simulink model "RequirementsTable"  (R2022b)
settings: Solver=FixedStepAuto  StartTime=0.0  StopTime=10.0  FixedStep=1e-3  RelTol=1e-3  EnableMultiTasking=on
settings Model: DVExtractedSubsystem=Requirements Table  Creator=TheCoaler  LastModifiedBy=TheCoaler
settings SolverCC: AlgebraicLoopSolver=TrustRegion
settings OptimizationCC: EnhancedBackFolding=on  PassReuseOutputArgsAs=Individual arguments  ZeroExternalMemoryAtStartup=off  ZeroInternalMemoryAtStartup=off  MaxStackSize=64  OptimizeBlockOrder=speed  DifferentSizesBufferReuse=on  OptimizationCustomize=off  EfficientTunableParamExpr=on
settings DebuggingCC: ParameterTunabilityLossMsg=error  UnconnectedInputMsg=warning  UnconnectedOutputMsg=warning  UnconnectedLineMsg=warning  FrameProcessingCompatibilityMsg=none  SFMachineParentedDataDiag=warning
settings HardwareCC: ProdBitPerPointer=32  ProdBitPerSizeT=32  ProdBitPerPtrDiffT=32  ProdLargestAtomicInteger=Long  ProdLargestAtomicFloat=Double  ProdWordSize=32  ProdHWDeviceType=ARM Compatible->ARM Cortex
settings ModelReferenceCC: EnableRefExpFcnMdlSchedulingChecks=on
settings SFSimCC: MATLABDynamicMemAlloc=off
settings RTWCC: Description=Embedded Coder  SystemTargetFile=ert.tlc  HardwareBoard=NXP FRDM-K64F  TemplateMakefile=ert_default_tmf  Toolchain=GNU Tools for ARM Embedded Processors
settings CodeAppCC: ForceParamTrailComments=on  IgnoreCustomStorageClasses=off  OperatorAnnotations=on  SimulinkDataObjDesc=on  SFDataObjDesc=on  InsertBlockDesc=on
settings ERTTargetCC: ExtMode=on  ExtModeTransport=4  ExtModeMexFile=sendToCommService  ExtModeMexArgs='RA_Modes' 0

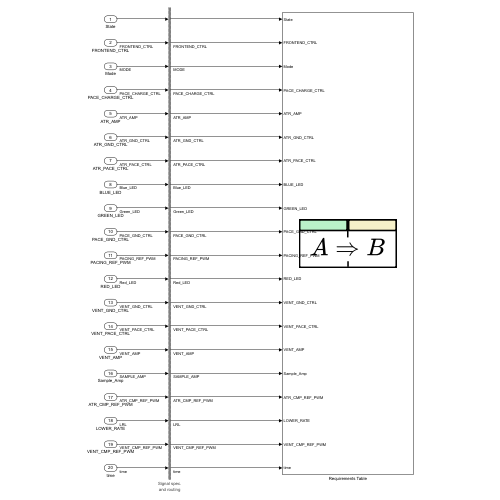
[thumbnail: Simulink's stored preview of the top-level diagram]
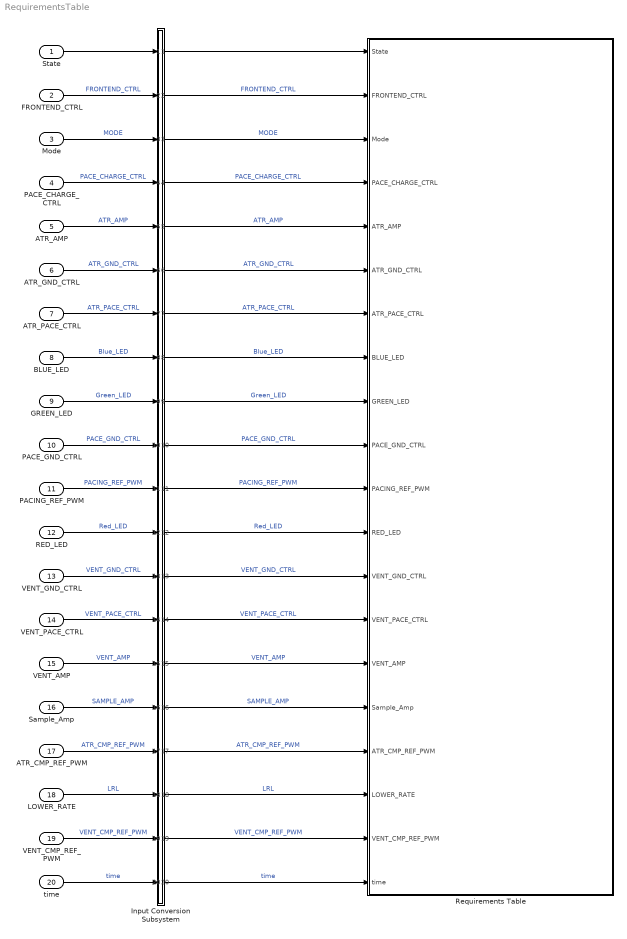
== system RequirementsTable ==
  State : Inport  OutDataTypeStr=boolean  PortDimensions=[1]  SampleTime=[-1, 0]  Interpolate=off
  FRONTEND_CTRL : Inport  Port=2  OutDataTypeStr=double  PortDimensions=[1]  SampleTime=0.001  Interpolate=off
  Mode : Inport  Port=3  OutDataTypeStr=double  PortDimensions=[1]  SampleTime=[-1, 0]  Interpolate=off
  PACE_CHARGE_CTRL : Inport  Port=4  OutDataTypeStr=double  PortDimensions=[1]  SampleTime=0.001  Interpolate=off
  ATR_AMP : Inport  Port=5  OutDataTypeStr=double  PortDimensions=[1]  SampleTime=[-1, 0]  Interpolate=off
  ATR_GND_CTRL : Inport  Port=6  OutDataTypeStr=double  PortDimensions=[1]  SampleTime=0.001  Interpolate=off
  ATR_PACE_CTRL : Inport  Port=7  OutDataTypeStr=double  PortDimensions=[1]  SampleTime=0.001  Interpolate=off
  BLUE_LED : Inport  Port=8  OutDataTypeStr=boolean  PortDimensions=[1]  SampleTime=0.001  Interpolate=off
  GREEN_LED : Inport  Port=9  OutDataTypeStr=boolean  PortDimensions=[1]  SampleTime=0.001  Interpolate=off
  PACE_GND_CTRL : Inport  Port=10  OutDataTypeStr=double  PortDimensions=[1]  SampleTime=0.001  Interpolate=off
  PACING_REF_PWM : Inport  Port=11  OutDataTypeStr=double  PortDimensions=[1]  SampleTime=0.001  Interpolate=off
  RED_LED : Inport  Port=12  OutDataTypeStr=boolean  PortDimensions=[1]  SampleTime=0.001  Interpolate=off
  VENT_GND_CTRL : Inport  Port=13  OutDataTypeStr=double  PortDimensions=[1]  SampleTime=0.001  Interpolate=off
  VENT_PACE_CTRL : Inport  Port=14  OutDataTypeStr=double  PortDimensions=[1]  SampleTime=0.001  Interpolate=off
  VENT_AMP : Inport  Port=15  OutDataTypeStr=double  PortDimensions=[1]  SampleTime=[-1, 0]  Interpolate=off
  Sample_Amp : Inport  Port=16  OutDataTypeStr=double  PortDimensions=[1]  SampleTime=[-1, 0]  Interpolate=off
  ATR_CMP_REF_PWM : Inport  Port=17  OutDataTypeStr=double  PortDimensions=[1]  SampleTime=0.001  Interpolate=off
  LOWER_RATE : Inport  Port=18  OutDataTypeStr=double  PortDimensions=[1]  SampleTime=[-1, 0]  Interpolate=off
  VENT_CMP_REF_PWM : Inport  Port=19  OutDataTypeStr=double  PortDimensions=[1]  SampleTime=0.001  Interpolate=off
  time : Inport  Port=20  OutDataTypeStr=double  PortDimensions=[1]  Interpolate=off
  Input Conversion Subsystem : Subsystem  Tag=__SLT_ICS__  Description=|
      | Signal spec.
      | and routing
      settings: AttributesFormatString=%<Description>
  Requirements Table : Requirements Table  TreatAsAtomicUnit=on
  wires:
  State/1 -> Input Conversion Subsystem/1(Inport_1)
  FRONTEND_CTRL/1 -> Input Conversion Subsystem/2(Inport_2)  "FRONTEND_CTRL"
  Mode/1 -> Input Conversion Subsystem/3(Inport_3)  "MODE"
  PACE_CHARGE_CTRL/1 -> Input Conversion Subsystem/4(Inport_4)  "PACE_CHARGE_CTRL"
  ATR_AMP/1 -> Input Conversion Subsystem/5(Inport_5)  "ATR_AMP"
  ATR_GND_CTRL/1 -> Input Conversion Subsystem/6(Inport_6)  "ATR_GND_CTRL"
  ATR_PACE_CTRL/1 -> Input Conversion Subsystem/7(Inport_7)  "ATR_PACE_CTRL"
  BLUE_LED/1 -> Input Conversion Subsystem/8(Inport_8)  "Blue_LED"
  GREEN_LED/1 -> Input Conversion Subsystem/9(Inport_9)  "Green_LED"
  PACE_GND_CTRL/1 -> Input Conversion Subsystem/10(Inport_10)  "PACE_GND_CTRL"
  PACING_REF_PWM/1 -> Input Conversion Subsystem/11(Inport_11)  "PACING_REF_PWM"
  RED_LED/1 -> Input Conversion Subsystem/12(Inport_12)  "Red_LED"
  VENT_GND_CTRL/1 -> Input Conversion Subsystem/13(Inport_13)  "VENT_GND_CTRL"
  VENT_PACE_CTRL/1 -> Input Conversion Subsystem/14(Inport_14)  "VENT_PACE_CTRL"
  VENT_AMP/1 -> Input Conversion Subsystem/15(Inport_15)  "VENT_AMP"
  Sample_Amp/1 -> Input Conversion Subsystem/16(Inport_16)  "SAMPLE_AMP"
  ATR_CMP_REF_PWM/1 -> Input Conversion Subsystem/17(Inport_17)  "ATR_CMP_REF_PWM"
  LOWER_RATE/1 -> Input Conversion Subsystem/18(Inport_18)  "LRL"
  VENT_CMP_REF_PWM/1 -> Input Conversion Subsystem/19(Inport_19)  "VENT_CMP_REF_PWM"
  time/1 -> Input Conversion Subsystem/20(Inport_20)  "time"
  Input Conversion Subsystem/1(Outport_1) -> Requirements Table/1(State)
  Input Conversion Subsystem/2(Outport_2) -> Requirements Table/2(FRONTEND_CTRL)  "FRONTEND_CTRL"
  Input Conversion Subsystem/3(Outport_3) -> Requirements Table/3(Mode)  "MODE"
  Input Conversion Subsystem/4(Outport_4) -> Requirements Table/4(PACE_CHARGE_CTRL)  "PACE_CHARGE_CTRL"
  Input Conversion Subsystem/5(Outport_5) -> Requirements Table/5(ATR_AMP)  "ATR_AMP"
  Input Conversion Subsystem/6(Outport_6) -> Requirements Table/6(ATR_GND_CTRL)  "ATR_GND_CTRL"
  Input Conversion Subsystem/7(Outport_7) -> Requirements Table/7(ATR_PACE_CTRL)  "ATR_PACE_CTRL"
  Input Conversion Subsystem/8(Outport_8) -> Requirements Table/8(BLUE_LED)  "Blue_LED"
  Input Conversion Subsystem/9(Outport_9) -> Requirements Table/9(GREEN_LED)  "Green_LED"
  Input Conversion Subsystem/10(Outport_10) -> Requirements Table/10(PACE_GND_CTRL)  "PACE_GND_CTRL"
  Input Conversion Subsystem/11(Outport_11) -> Requirements Table/11(PACING_REF_PWM)  "PACING_REF_PWM"
  Input Conversion Subsystem/12(Outport_12) -> Requirements Table/12(RED_LED)  "Red_LED"
  Input Conversion Subsystem/13(Outport_13) -> Requirements Table/13(VENT_GND_CTRL)  "VENT_GND_CTRL"
  Input Conversion Subsystem/14(Outport_14) -> Requirements Table/14(VENT_PACE_CTRL)  "VENT_PACE_CTRL"
  Input Conversion Subsystem/15(Outport_15) -> Requirements Table/15(VENT_AMP)  "VENT_AMP"
  Input Conversion Subsystem/16(Outport_16) -> Requirements Table/16(Sample_Amp)  "SAMPLE_AMP"
  Input Conversion Subsystem/17(Outport_17) -> Requirements Table/17(ATR_CMP_REF_PWM)  "ATR_CMP_REF_PWM"
  Input Conversion Subsystem/18(Outport_18) -> Requirements Table/18(LOWER_RATE)  "LRL"
  Input Conversion Subsystem/19(Outport_19) -> Requirements Table/19(VENT_CMP_REF_PWM)  "VENT_CMP_REF_PWM"
  Input Conversion Subsystem/20(Outport_20) -> Requirements Table/20(time)  "time"

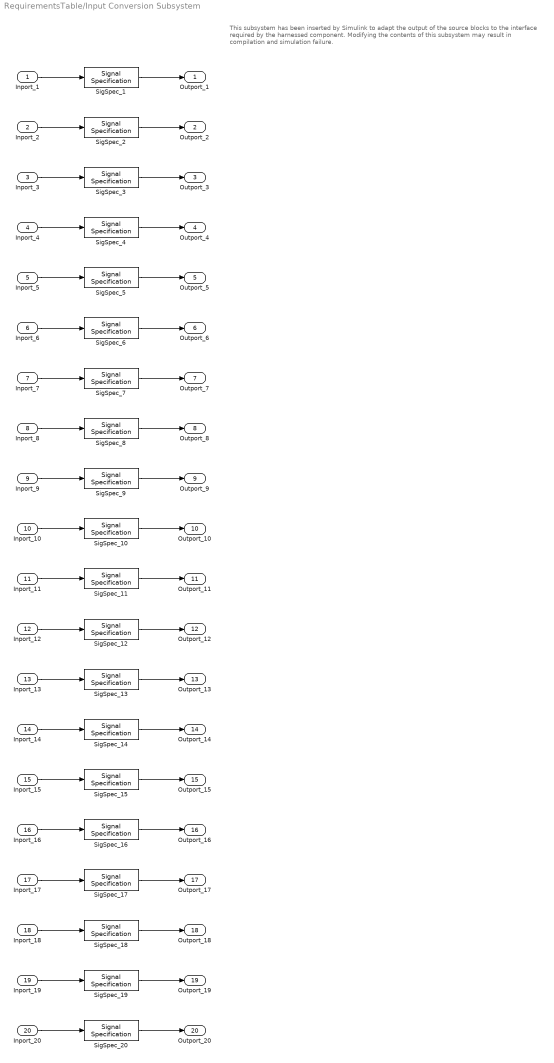
== system RequirementsTable/Input Conversion Subsystem ==
  note: This subsystem has been inserted by Simulink to adapt the output of the source blocks to the interface required by the harnessed component.
      |  Modifying the contents of this subsystem may result in compilation and simulation failure.
  Inport_1 : Inport
  Inport_2 : Inport  Port=2
  Inport_3 : Inport  Port=3
  Inport_4 : Inport  Port=4
  Inport_5 : Inport  Port=5
  Inport_6 : Inport  Port=6
  Inport_7 : Inport  Port=7
  Inport_8 : Inport  Port=8
  Inport_9 : Inport  Port=9
  Inport_10 : Inport  Port=10
  Inport_11 : Inport  Port=11
  Inport_12 : Inport  Port=12
  Inport_13 : Inport  Port=13
  Inport_14 : Inport  Port=14
  Inport_15 : Inport  Port=15
  Inport_16 : Inport  Port=16
  Inport_17 : Inport  Port=17
  Inport_18 : Inport  Port=18
  Inport_19 : Inport  Port=19
  Inport_20 : Inport  Port=20
  SigSpec_1 : SignalSpecification  OutDataTypeStr=boolean  Dimensions=[1]  SampleTime=[-1, 0]
  SigSpec_{2,4,6..7,10..11,13..14,17,19} (10 alike) : SignalSpecification  OutDataTypeStr=double  Dimensions=[1]  SampleTime=0.001
  SigSpec_12 : SignalSpecification  OutDataTypeStr=boolean  Dimensions=[1]  SampleTime=0.001
  SigSpec_{3,5,15..16,18} (5 alike) : SignalSpecification  OutDataTypeStr=double  Dimensions=[1]  SampleTime=[-1, 0]
  SigSpec_20 : SignalSpecification  OutDataTypeStr=double  Dimensions=[1]
  SigSpec_8 : SignalSpecification  OutDataTypeStr=boolean  Dimensions=[1]  SampleTime=0.001
  SigSpec_9 : SignalSpecification  OutDataTypeStr=boolean  Dimensions=[1]  SampleTime=0.001
  Outport_1 : Outport
  Outport_2 : Outport  Port=2
  Outport_3 : Outport  Port=3
  Outport_4 : Outport  Port=4
  Outport_5 : Outport  Port=5
  Outport_6 : Outport  Port=6
  Outport_7 : Outport  Port=7
  Outport_8 : Outport  Port=8
  Outport_9 : Outport  Port=9
  Outport_10 : Outport  Port=10
  Outport_11 : Outport  Port=11
  Outport_12 : Outport  Port=12
  Outport_13 : Outport  Port=13
  Outport_14 : Outport  Port=14
  Outport_15 : Outport  Port=15
  Outport_16 : Outport  Port=16
  Outport_17 : Outport  Port=17
  Outport_18 : Outport  Port=18
  Outport_19 : Outport  Port=19
  Outport_20 : Outport  Port=20
  wires:
  SigSpec_1/1 -> Outport_1/1
  Inport_1/1 -> SigSpec_1/1
  SigSpec_2/1 -> Outport_2/1
  Inport_2/1 -> SigSpec_2/1
  SigSpec_3/1 -> Outport_3/1
  Inport_3/1 -> SigSpec_3/1
  SigSpec_4/1 -> Outport_4/1
  Inport_4/1 -> SigSpec_4/1
  SigSpec_5/1 -> Outport_5/1
  Inport_5/1 -> SigSpec_5/1
  SigSpec_6/1 -> Outport_6/1
  Inport_6/1 -> SigSpec_6/1
  SigSpec_7/1 -> Outport_7/1
  Inport_7/1 -> SigSpec_7/1
  SigSpec_8/1 -> Outport_8/1
  Inport_8/1 -> SigSpec_8/1
  SigSpec_9/1 -> Outport_9/1
  Inport_9/1 -> SigSpec_9/1
  SigSpec_10/1 -> Outport_10/1
  Inport_10/1 -> SigSpec_10/1
  SigSpec_11/1 -> Outport_11/1
  Inport_11/1 -> SigSpec_11/1
  SigSpec_12/1 -> Outport_12/1
  Inport_12/1 -> SigSpec_12/1
  SigSpec_13/1 -> Outport_13/1
  Inport_13/1 -> SigSpec_13/1
  SigSpec_14/1 -> Outport_14/1
  Inport_14/1 -> SigSpec_14/1
  SigSpec_15/1 -> Outport_15/1
  Inport_15/1 -> SigSpec_15/1
  SigSpec_16/1 -> Outport_16/1
  Inport_16/1 -> SigSpec_16/1
  SigSpec_17/1 -> Outport_17/1
  Inport_17/1 -> SigSpec_17/1
  SigSpec_18/1 -> Outport_18/1
  Inport_18/1 -> SigSpec_18/1
  SigSpec_19/1 -> Outport_19/1
  Inport_19/1 -> SigSpec_19/1
  SigSpec_20/1 -> Outport_20/1
  Inport_20/1 -> SigSpec_20/1

== stateflow chart RequirementsTable/Requirements Table ==
  (default) -> (junction 1073748699)
  (junction 1073748699) -> (junction 1073748700) : {
      | % SF_REQ_REV_07
      | }
  (junction 1073748700) -> (junction 1073748702) : {
      | % HEADER_ASSIGNMENTS
      |
      | }
  (junction 1073748702) -> (junction 1073748912) : {
      | % START_A_28
      | }
  (junction 1073748912) -> (junction 1073748914) : {
      | }
  (junction 1073748914) -> (junction 1073748916) : {
      | reqtable_assumption((Mode<=4), 28);
      | }
  (junction 1073748916) -> (junction 1073748918) : {
      | }
  (junction 1073748918) -> (junction 1073749000) : {
      | % START_A_130
      | }
  (junction 1073749000) -> (junction 1073749002) : {
      | }
  (junction 1073749002) -> (junction 1073749004) : {
      | reqtable_assumption((Mode>=1), 130);
      | }
  (junction 1073749004) -> (junction 1073749006) : {
      | }
  (junction 1073749006) -> (junction 1073749008) : {
      | % END_A_130
      | }
  (junction 1073749008) -> (junction 1073749012) : {
      | % START_A_139
      | }
  (junction 1073749012) -> (junction 1073749014) : {
      | }
  (junction 1073749014) -> (junction 1073749016) : {
      | reqtable_assumption((rem(Mode,1)==0), 139);
      | }
  (junction 1073749016) -> (junction 1073749018) : {
      | }
  (junction 1073749018) -> (junction 1073749056) : {
      | % END_A_139
      | }
  (junction 1073749056) -> (junction 1073748930) : {
      | % END_A_28
      | }
  (junction 1073748930) -> (junction 1073748934) : {
      | % START_A_106
      | }
  (junction 1073748934) -> (junction 1073748936) : {
      | }
  (junction 1073748936) -> (junction 1073748938) : {
      | reqtable_assumption((State<=1), 106);
      | }
  (junction 1073748938) -> (junction 1073748940) : {
      | }
  (junction 1073748940) -> (junction 1073748942) : {
      | % START_A_133
      | }
  (junction 1073748942) -> (junction 1073748944) : {
      | }
  (junction 1073748944) -> (junction 1073748946) : {
      | reqtable_assumption((State>=0), 133);
      | }
  (junction 1073748946) -> (junction 1073748948) : {
      | }
  (junction 1073748948) -> (junction 1073748950) : {
      | % END_A_133
      | }
  (junction 1073748950) -> (junction 1073748952) : {
      | % END_A_106
      | }
  (junction 1073748952) -> (junction 1073748956) : {
      | % START_A_109
      | }
  (junction 1073748956) -> (junction 1073748958) : {
      | }
  (junction 1073748958) -> (junction 1073748960) : {
      | reqtable_assumption((FRONTEND_CTRL<=1), 109);
      | }
  (junction 1073748960) -> (junction 1073748962) : {
      | }
  (junction 1073748962) -> (junction 1073748964) : {
      | % START_A_136
      | }
  (junction 1073748964) -> (junction 1073748966) : {
      | }
  (junction 1073748966) -> (junction 1073748968) : {
      | reqtable_assumption((FRONTEND_CTRL>=0), 136);
      | }
  (junction 1073748968) -> (junction 1073748970) : {
      | }
  (junction 1073748970) -> (junction 1073748972) : {
      | % END_A_136
      | }
  (junction 1073748972) -> (junction 1073748974) : {
      | % END_A_109
      | }
  (junction 1073748974) -> (junction 1073749060) : {
      | % START_A_151
      | }
  (junction 1073749060) -> (junction 1073749062) : {
      | }
  (junction 1073749062) -> (junction 1073749064) : {
      | reqtable_assumption((time>0), 151);
      | }
  (junction 1073749064) -> (junction 1073749066) : {
      | }
  (junction 1073749066) -> (junction 1073749068) : {
      | % END_A_151
      | }
  (junction 1073749068) -> (junction 1073748734) : {
      | % START_R_1
      | }
  (junction 1073748734) -> (junction 1073748736) : {
      | }
  (junction 1073748736) -> (junction 1073748738)
  (junction 1073748738) -> (junction 1073748740) [order 1] : [(((Mode) == (1))) && (((State) == (0)))]
  (junction 1073748738) -> (junction 1073748746) [order 2]
  (junction 1073748740) -> (junction 1073748742) : {
      | reqtable_postcondition((((PACE_CHARGE_CTRL) == (1))) && (ATR_PACE_CTRL == 0) && (((PACING_REF_PWM ) == (ATR_AMP))) && (((PACE_CHARGE_CTRL) == (1))) && (((PACE_GND_CTRL) == (1))) && (ATR_GND_CTRL == 1) && (((RED_LED) == (0))) && (((GREEN_LED) == (0))) && (((BLUE_LED) == (0))) && (time-oldTime / (60*1000) >= LOWER_RATE), 'R:1');
      |
      | }
  (junction 1073748742) -> (junction 1073748744) : {
      | }
  (junction 1073748744) -> (junction 1073748746)
  (junction 1073748746) -> (junction 1073748748)
  (junction 1073748748) -> (junction 1073748750) : {
      | % END_R_1
      | }
  (junction 1073748750) -> (junction 1073748752) : {
      | % START_R_7
      | }
  (junction 1073748752) -> (junction 1073748754) : {
      | }
  (junction 1073748754) -> (junction 1073748756)
  (junction 1073748756) -> (junction 1073748758) [order 1] : [(((Mode) == (1))) && (((State) == (1)))]
  (junction 1073748756) -> (junction 1073748764) [order 2]
  (junction 1073748758) -> (junction 1073748760) : {
      | reqtable_postcondition((((PACE_CHARGE_CTRL) == (0))) && (ATR_PACE_CTRL == 1) && (((PACING_REF_PWM ) == (ATR_AMP))) && (((PACE_CHARGE_CTRL) == (0))) && (((PACE_GND_CTRL) == (1))) && (ATR_GND_CTRL == 0) && (((RED_LED) == (1))) && (((GREEN_LED) == (0))) && (((BLUE_LED) == (0))) && (time-oldTime / (60*1000) >= LOWER_RATE), 'R:2');
      |
      | }
  (junction 1073748760) -> (junction 1073748762) : {
      | }
  (junction 1073748762) -> (junction 1073748764)
  (junction 1073748764) -> (junction 1073748766)
  (junction 1073748766) -> (junction 1073748768) : {
      | % END_R_7
      | }
  (junction 1073748768) -> (junction 1073748770) : {
      | % START_R_10
      | }
  (junction 1073748770) -> (junction 1073748772) : {
      | }
  (junction 1073748772) -> (junction 1073748774)
  (junction 1073748774) -> (junction 1073748776) [order 1] : [(((Mode) == (3))) && (((State) == (0)))]
  (junction 1073748774) -> (junction 1073748782) [order 2]
  (junction 1073748776) -> (junction 1073748778) : {
      | reqtable_postcondition((((PACE_CHARGE_CTRL) == (1))) && (VENT_PACE_CTRL == 0) && (((PACING_REF_PWM ) == (VENT_AMP))) && (((PACE_CHARGE_CTRL) == (1))) && (((PACE_GND_CTRL) == (1))) && (VENT_GND_CTRL == 1) && (((RED_LED) == (0))) && (((GREEN_LED) == (0))) && (((BLUE_LED) == (0))) && (time-oldTime / (60*1000) >= LOWER_RATE), 'R:3');
      |
      | }
  (junction 1073748778) -> (junction 1073748780) : {
      | }
  (junction 1073748780) -> (junction 1073748782)
  (junction 1073748782) -> (junction 1073748784)
  (junction 1073748784) -> (junction 1073748786) : {
      | % END_R_10
      | }
  (junction 1073748786) -> (junction 1073748788) : {
      | % START_R_13
      | }
  (junction 1073748788) -> (junction 1073748790) : {
      | }
  (junction 1073748790) -> (junction 1073748792)
  (junction 1073748792) -> (junction 1073748794) [order 1] : [(((Mode) == (3))) && (((State) == (1)))]
  (junction 1073748792) -> (junction 1073748800) [order 2]
  (junction 1073748794) -> (junction 1073748796) : {
      | reqtable_postcondition((((PACE_CHARGE_CTRL) == (0))) && (VENT_PACE_CTRL == 1) && (((PACING_REF_PWM ) == (VENT_AMP))) && (((PACE_CHARGE_CTRL) == (0))) && (((PACE_GND_CTRL) == (1))) && (VENT_GND_CTRL == 0) && (((RED_LED) == (0))) && (((GREEN_LED) == (1))) && (((BLUE_LED) == (0))) && (time-oldTime / (60*1000) >= LOWER_RATE), 'R:4');
      |
      | }
  (junction 1073748796) -> (junction 1073748798) : {
      | }
  (junction 1073748798) -> (junction 1073748800)
  (junction 1073748800) -> (junction 1073748802)
  (junction 1073748802) -> (junction 1073748804) : {
      | % END_R_13
      | }
  (junction 1073748804) -> (junction 1073748806) : {
      | % START_R_16
      | }
  (junction 1073748806) -> (junction 1073748808) : {
      | }
  (junction 1073748808) -> (junction 1073748810)
  (junction 1073748810) -> (junction 1073748812) [order 1] : [(((Mode) == (2))) && (((State) == (0))) && (FRONTEND_CTRL == 1)]
  (junction 1073748810) -> (junction 1073748818) [order 2]
  (junction 1073748812) -> (junction 1073748814) : {
      | reqtable_postcondition((((PACE_CHARGE_CTRL) == (1))) && (ATR_PACE_CTRL == 0) && (((PACING_REF_PWM ) == (ATR_AMP))) && (((PACE_CHARGE_CTRL) == (1))) && (((PACE_GND_CTRL) == (1))) && (ATR_GND_CTRL == 1) && (((RED_LED) == (0))) && (((GREEN_LED) == (0))) && (((BLUE_LED) == (0))) && (ATR_CMP_REF_PWM == Sample_Amp) && (time-oldTime / (60*1000) >= LOWER_RATE), 'R:5');
      |
      | }
  (junction 1073748814) -> (junction 1073748816) : {
      | }
  (junction 1073748816) -> (junction 1073748818)
  (junction 1073748818) -> (junction 1073748820)
  (junction 1073748820) -> (junction 1073748822) : {
      | % END_R_16
      | }
  (junction 1073748822) -> (junction 1073748824) : {
      | % START_R_19
      | }
  (junction 1073748824) -> (junction 1073748826) : {
      | }
  (junction 1073748826) -> (junction 1073748828)
  (junction 1073748828) -> (junction 1073748830) [order 1] : [(((Mode) == (2))) && (((State) == (1)))]
  (junction 1073748828) -> (junction 1073748836) [order 2]
  (junction 1073748830) -> (junction 1073748832) : {
      | reqtable_postcondition((((PACE_CHARGE_CTRL) == (0))) && (ATR_PACE_CTRL == 1) && (((PACING_REF_PWM ) == (ATR_AMP))) && (((PACE_CHARGE_CTRL) == (0))) && (((PACE_GND_CTRL) == (1))) && (ATR_GND_CTRL == 0) && (((RED_LED) == (0))) && (((GREEN_LED) == (0))) && (((BLUE_LED) == (0))) && (ATR_CMP_REF_PWM == Sample_Amp) && (time-oldTime / (60*1000) >= LOWER_RATE), 'R:6');
      |
      | }
  (junction 1073748832) -> (junction 1073748834) : {
      | }
  (junction 1073748834) -> (junction 1073748836)
  (junction 1073748836) -> (junction 1073748838)
  (junction 1073748838) -> (junction 1073748840) : {
      | % END_R_19
      | }
  (junction 1073748840) -> (junction 1073748842) : {
      | % START_R_22
      | }
  (junction 1073748842) -> (junction 1073748844) : {
      | }
  (junction 1073748844) -> (junction 1073748846)
  (junction 1073748846) -> (junction 1073748848) [order 1] : [(((Mode) == (4))) && (((State) == (0))) && (FRONTEND_CTRL == 1)]
  (junction 1073748846) -> (junction 1073748854) [order 2]
  (junction 1073748848) -> (junction 1073748850) : {
      | reqtable_postcondition((((PACE_CHARGE_CTRL) == (1))) && (VENT_PACE_CTRL == 0) && (((PACING_REF_PWM ) == (VENT_AMP))) && (((PACE_CHARGE_CTRL) == (1))) && (((PACE_GND_CTRL) == (1))) && (VENT_GND_CTRL == 1) && (((RED_LED) == (0))) && (((GREEN_LED) == (0))) && (((BLUE_LED) == (0))) && (VENT_CMP_REF_PWM == Sample_Amp) && (time-oldTime / (60*1000) >= LOWER_RATE), 'R:7');
      |
      | }
  (junction 1073748850) -> (junction 1073748852) : {
      | }
  (junction 1073748852) -> (junction 1073748854)
  (junction 1073748854) -> (junction 1073748856)
  (junction 1073748856) -> (junction 1073748858) : {
      | % END_R_22
      | }
  (junction 1073748858) -> (junction 1073748860) : {
      | % START_R_25
      | }
  (junction 1073748860) -> (junction 1073748862) : {
      | }
  (junction 1073748862) -> (junction 1073748864)
  (junction 1073748864) -> (junction 1073748866) [order 1] : [(((Mode) == (4))) && (((State) == (1)))]
  (junction 1073748864) -> (junction 1073748872) [order 2]
  (junction 1073748866) -> (junction 1073748868) : {
      | reqtable_postcondition((((PACE_CHARGE_CTRL) == (0))) && (VENT_PACE_CTRL == 1) && (((PACING_REF_PWM ) == (VENT_AMP))) && (((PACE_CHARGE_CTRL) == (0))) && (((PACE_GND_CTRL) == (1))) && (VENT_GND_CTRL == 0) && (((RED_LED) == (0))) && (((GREEN_LED) == (1))) && (((BLUE_LED) == (0))) && (VENT_CMP_REF_PWM == Sample_Amp) && (time-oldTime / (60*1000) >= LOWER_RATE), 'R:8');
      |
      | }
  (junction 1073748868) -> (junction 1073748870) : {
      | }
  (junction 1073748870) -> (junction 1073748872)
  (junction 1073748872) -> (junction 1073748874)
  (junction 1073748874) -> (junction 1073748876) : {
      | % END_R_25
      | }
  data: State input; FRONTEND_CTRL input; Mode input; PACE_CHARGE_CTRL input; ATR_AMP input; ATR_GND_CTRL input; ATR_PACE_CTRL input; BLUE_LED input; GREEN_LED input; PACE_GND_CTRL input; PACING_REF_PWM input; RED_LED input; VENT_GND_CTRL input; VENT_PACE_CTRL input; VENT_AMP input; Sample_Amp input; ATR_CMP_REF_PWM input; LOWER_RATE input; VENT_CMP_REF_PWM input; time input [0..]; oldTime constant double =0
